simulink model "productionLine_5machines"  (R2024b)
settings: Solver=ode15s  StartTime=0.0  StopTime=100  FixedStep=0.1  RelTol=1e-3
model workspace (MAT data in the model file):
  bufferCapacity1 = 50
  bufferCapacity2 = 50
  bufferCapacity3 = 50
  bufferCapacity4 = 50
  bufferProcessedProducts = 50
  initialBufferCapacity = 100
undefined symbols (not defined in the file): m, n
libraries: rllib x1
settings Model: SimulationMode=accelerator  Creator=giopa  LastModifiedBy=giopa

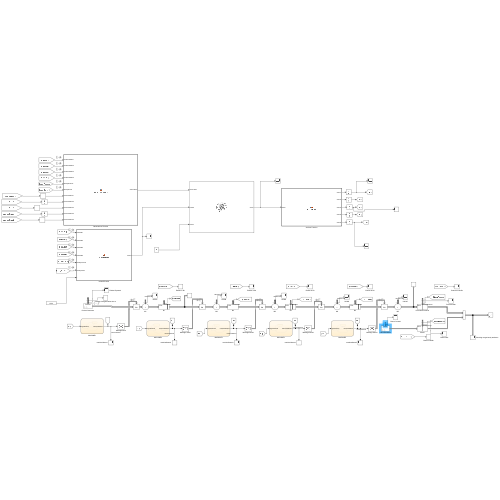
[thumbnail: Simulink's stored preview of the top-level diagram]
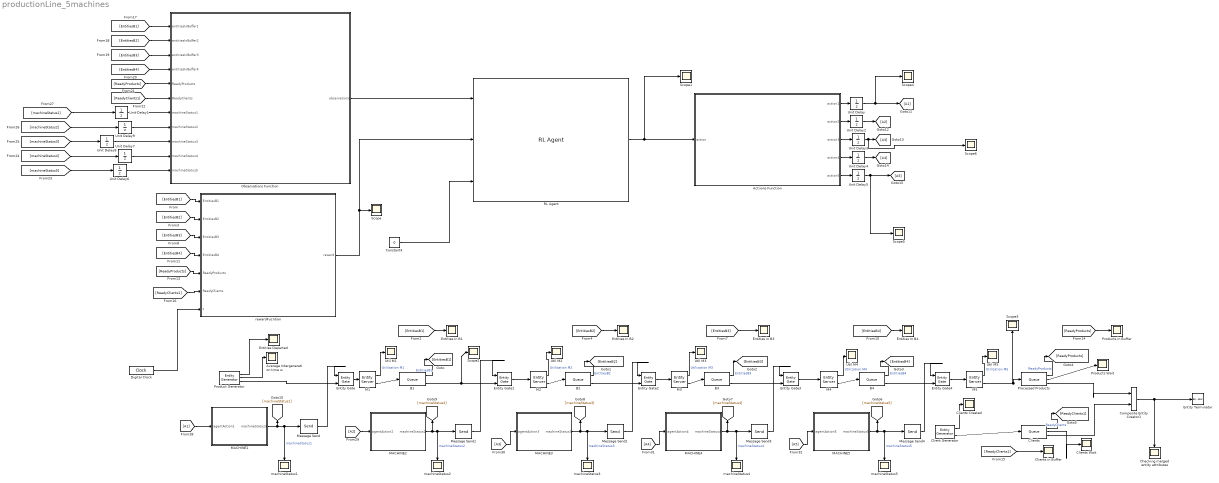
== system productionLine_5machines ==
  Actiions Function : MATLAB Function  TreatAsAtomicUnit=on
  Average Intergeneration time w : Scope
  B1 : Queue  InputPortMessageModes=m  OutputPortMessageModes=n,m  Capacity=bufferCapacity1  NumberEntitiesInBlock=on
      settings: OutputPortMap=o1,o5
  B2 : Queue  InputPortMessageModes=m  OutputPortMessageModes=n,m  Capacity=bufferCapacity2  NumberEntitiesInBlock=on
      settings: OutputPortMap=o1,o5
  B3 : Queue  InputPortMessageModes=m  OutputPortMessageModes=n,m  Capacity=bufferCapacity3  NumberEntitiesInBlock=on
      settings: OutputPortMap=o1,o5
  B4 : Queue  InputPortMessageModes=m  OutputPortMessageModes=n,m  Capacity=bufferCapacity4  NumberEntitiesInBlock=on
      settings: OutputPortMap=o1,o5
  Checking merged entity attributes : Scope
  Client Generator : EntityGenerator  OutputPortMessageModes=n,m  TimeSource=MATLAB action  IntergenerationTimeAction=|  GenerateEntityAtSimulationStart=off  GenerateAction=|  AttributeName=clientNumber  NumberEntitiesDeparted=on  EntityType=Structured  EntityTypeName=Client
      IntergenerationTimeAction=|
      | muI = 4.5;   % Mean intergeneration time 
      | dt = -muI * log(1 - rand());  % Exponential distribution
      GenerateAction=|
      | persistent clientNumber;
      | if isempty(clientNumber)
      |     clientNumber = 0; % Initialize the first client number
      | else
      |     clientNumber = clientNumber + 1; % Increment client number for each new entity
      | end
      | entity.clientNumber = clientNumber; % Assign the number to the entity's attribute
      settings: OutputPortMap=o0,o3
  "Clients " : Queue  InputPortMessageModes=m  OutputPortMessageModes=n,n,m  Capacity=50  NumberEntitiesInBlock=on  AverageWait=on
      settings: OutputPortMap=o1,o2,o5
  Clients Created : Scope
  Clients Wait : Scope
  Clients in Buffer : Scope
  Composite Entity Creator1 : CompositeEntityCreator  InputPortMessageModes=m,m  OutputPortMessageModes=m  EntityTypeName=Order  InputEntityName=Product|Client
      settings: InputPortMap=u0,u1
  Constant4 : Constant  Value=0
  Digital Clock : DigitalClock  SampleTime=0.1
  Entities Departed : Scope
  Entities In B1 : Scope
  Entities In B2 : Scope
  Entities In B4 : Scope
  Entities in B3 : Scope
  Entity Gate : EntityGate  InputPortMessageModes=m,m  OutputPortMessageModes=m  MatchingAttributeName=gateCheck  InitialValueOfMatchingAttribute=1  OpenGateAtSimulationStart=on
  Entity Gate{1..4} (4 alike) : EntityGate  InputPortMessageModes=m,m  OutputPortMessageModes=m  MatchingAttributeName=machineStatus  InitialValueOfMatchingAttribute=1
  Entity Terminator : EntityTerminator  InputPortMessageModes=m
  M{1..5} (5 alike) : EntityServer  InputPortMessageModes=m  OutputPortMessageModes=n,m  Capacity=1  ServiceTimeSource=Attribute  ServiceTimeValue=1  ServiceTimeAttributeName=processingTime  Utilization=on
      settings: OutputPortMap=o5,o9
  MACHINE1 : Stateflow chart  TreatAsAtomicUnit=on
  MACHINE2 : Stateflow chart  TreatAsAtomicUnit=on
  MACHINE3 : Stateflow chart  TreatAsAtomicUnit=on
  MACHINE4 : Stateflow chart  TreatAsAtomicUnit=on
  MACHINE5 : Stateflow chart  TreatAsAtomicUnit=on
  Message Send{,1..4} (5 alike) : Send  OutputPortMessageModes=m
  Observations Function : MATLAB Function  TreatAsAtomicUnit=on
  Processed Products : Queue  InputPortMessageModes=m  OutputPortMessageModes=n,n,m  Capacity=bufferProcessedProducts  NumberEntitiesInBlock=on  AverageWait=on
      settings: OutputPortMap=o1,o2,o5
  Product Generator : EntityGenerator  OutputPortMessageModes=n,n,m  Period=2.7  IntergenerationTimeAction=|  GenerateAction=|  ExitAction=|  AttributeName=processingTime|productNumber|entryTime  AttributeInitialValue=2|1|1  NumberEntitiesDeparted=on  AverageIntergenerationTime=on  EntityType=Structured  EntityTypeName=Product
      IntergenerationTimeAction=|
      | muI = 2;   % Mean intergeneration time 
      | dt = -muI * log(1 - rand());  % Exponential distribution
      GenerateAction=|
      | persistent rngInit;
      | if isempty(rngInit)
      |     seed = 12345;
      |     rng(seed);
      |     rngInit = true;
      | end
      | % Pattern: Exponential distribution
      | 
      | mu = 2;
      | entity.processingTime = -mu * log(1 - rand());
      | 
      | %assign productNumber aatribute to every entity
      | persistent productNumber
      | if isempty(productNumber)
      |     productNumber = 0;  
      | end
      | 
      | % Assign productNumber attribute
      | entity.productNumber = productNumber + 1; % Increment and assign the product number
      | productNumber = productNumber + 1;        % Update the product number for the next product
      ExitAction=|
      | persistent productNumber;
      | if isempty(productNumber)
      |     productNumber = 1; % Initialize the first client number
      | else
      |     productNumber = productNumber + 1; % Increment client number for each new entity
      | end
      | entity.productNumber = productNumber; % Assign the number to the entity's attribute
      settings: OutputPortMap=o0,o2,o3
  Products Wait : Scope
  Products in Buffer : Scope
  RL Agent : rllib/RL Agent  Agent=agent  ExternalActionAsInput=off  ProvideLastAction=off  ProvideCumRwd=off  TreatAsDirectFeedthrough=on  UseStrictObservationDataTypes=off
  Scope{,1..6} (7 alike) : Scope
  Unit Delay{,2..5} (5 alike) : UnitDelay  SampleTime=-1  HasFrameUpgradeWarning=on
  Unit Delay{1,6..9} (5 alike) : UnitDelay  InitialCondition=1  SampleTime=-1  HasFrameUpgradeWarning=on
  Util M{1..5} (5 alike) : Scope
  machineStatus{1..5} (5 alike) : Scope
  rewardFucntion : MATLAB Function  TreatAsAtomicUnit=on
  wires:
  Processed Products/2 -> Products Wait/1
  Entity Gate4/1 -> M5/1
  Product Generator/3 -> Entity Gate/2
  MACHINE3/1(machineStatus3) -> Message Send2/1, machineStatus3/1, [machineStatus3]  "machineStatus3"
  M1/1 -> Util M1/1  "Utilization M1"
  MACHINE1/1(machineStatus1) -> machineStatus1/1, Message Send/1, [machineStatus1]  "machineStatus1"
  MACHINE4/1(machineStatus4) -> Message Send3/1, machineStatus4/1, [machineStatus4]  "machineStatus4"
  MACHINE5/1(machineStatus5) -> Message Send4/1, machineStatus5/1, [machineStatus5]  "machineStatus5"
  B1/2 -> Scope2/1, Entity Gate1/2
  "Clients "/2 -> Clients Wait/1
  Product Generator/2 -> Average Intergeneration time w/1
  Processed Products/3 -> Composite Entity Creator1/1
  Client Generator/2 -> "Clients "/1
  M2/1 -> Util M2/1  "Utilization M2"
  Message Send3/1 -> Entity Gate3/1
  M4/1 -> Util M4/1  "Utilization M4"
  "Clients "/3 -> Composite Entity Creator1/2
  Entity Gate3/1 -> M4/1
  Entity Gate1/1 -> M2/1
  Entity Gate/1 -> M1/1
  Product Generator/1 -> Entities Departed/1
  M5/1 -> Util M5/1  "Utilization M5"
  Client Generator/1 -> Clients Created/1
  Composite Entity Creator1/1 -> Entity Terminator/1, Checking merged entity attributes/1
  B4/2 -> Entity Gate4/2
  M3/2 -> B3/1
  MACHINE2/1(machineStatus2) -> [machineStatus2], machineStatus2/1, Message Send1/1  "machineStatus2"
  Message Send2/1 -> Entity Gate2/1
  M3/1 -> Util M3/1  "Utilization M3"
  M4/2 -> B4/1
  B2/2 -> Entity Gate2/2
  Entity Gate2/1 -> M3/1
  Message Send4/1 -> Entity Gate4/1
  Message Send1/1 -> Entity Gate1/1
  M5/2 -> Processed Products/1, Scope3/1
  B3/2 -> Entity Gate3/2
  M2/2 -> B2/1
  Message Send/1 -> Entity Gate/1
  rewardFucntion/1(reward) -> Scope/1, RL Agent/2
  M1/2 -> B1/1
  B1/1 -> [EntitiesB1]  "EntitiesB1"
  [EntitiesB1] -> rewardFucntion/1(EntitiesB1)
  [EntitiesB1] -> Entities In B1/1
  B2/1 -> [EntitiesB2]  "EntitiesB2"
  [EntitiesB2] -> rewardFucntion/2(EntitiesB2)
  [EntitiesB2] -> Entities In B2/1
  B3/1 -> [EntitiesB3]  "EntitiesB3"
  [EntitiesB3] -> rewardFucntion/3(EntitiesB3)
  B4/1 -> [EntitiesB4]  "EntitiesB4"
  [EntitiesB4] -> Entities In B4/1
  [EntitiesB4] -> rewardFucntion/4(EntitiesB4)
  Processed Products/1 -> [ReadyProducts]  "ReadyProducts"
  [ReadyProducts] -> rewardFucntion/5(ReadyProducts)
  [ReadyProducts] -> Products in Buffer/1
  [ReadyClients1] -> rewardFucntion/6(ReadyClients)
  [EntitiesB3] -> Entities in B3/1
  [EntitiesB1] -> Observations Function/1(entitiesInBuffer1)
  [EntitiesB2] -> Observations Function/2(entitiesInBuffer2)
  [EntitiesB3] -> Observations Function/3(entitiesInBuffer3)
  "Clients "/1 -> [ReadyClients1]  "ReadyClients"
  [ReadyClients1] -> Clients in Buffer/1
  [ReadyProducts] -> Observations Function/5(ReadyProducts)
  [ReadyClients1] -> Observations Function/6(ReadyClients)
  [EntitiesB4] -> Observations Function/4(entitiesInBuffer4)
  [machineStatus5] -> Unit Delay6/1
  [machineStatus4] -> Unit Delay7/1
  [machineStatus3] -> Unit Delay8/1
  [machineStatus2] -> Unit Delay9/1
  [machineStatus1] -> Unit Delay1/1
  Observations Function/1(observations) -> RL Agent/1
  Constant4/1 -> RL Agent/3
  RL Agent/1 -> Scope1/1, Actiions Function/1(action)
  Actiions Function/1(action1) -> Unit Delay/1
  [A1] -> MACHINE1/1(agentAction1)
  Actiions Function/2(action2) -> Unit Delay2/1
  [A2] -> MACHINE2/1(agentAction2)
  Actiions Function/3(action3) -> Unit Delay3/1
  [A3] -> MACHINE3/1(agentAction3)
  Actiions Function/4(action4) -> Unit Delay4/1
  [A4] -> MACHINE4/1(agentAction4)
  Actiions Function/5(action5) -> Unit Delay5/1
  [A5] -> MACHINE5/1(agentAction5)
  Unit Delay/1 -> Scope4/1, [A1]
  Unit Delay1/1 -> Observations Function/7(machineStatus1)
  Unit Delay2/1 -> [A2]
  Unit Delay3/1 -> Scope6/1, [A3]
  Unit Delay4/1 -> [A4]
  Unit Delay5/1 -> Scope5/1, [A5]
  Unit Delay6/1 -> Observations Function/11(machineStatus5)
  Unit Delay7/1 -> Observations Function/10(machineStatus4)
  Unit Delay8/1 -> Observations Function/9(machineStatus3)
  Unit Delay9/1 -> Observations Function/8(machineStatus2)
  Digital Clock/1 -> rewardFucntion/7(t)

== stateflow chart productionLine_5machines/MACHINE5 ==
  state Failed
    entry:
    machineStatus5 = 0;
    repairTime5 = -meanRepairTime5 * log(1 - rand());
  state Idle
    entry:
    machineStatus5 = -1;
  state Working
    entry:
    machineStatus5 = 1;
    timeToFailure5 = -meanFailureTime5 * log(1 - rand());
  Working -> Failed [order 1] : [after(timeToFailure5, sec)]
  Failed -> Working : [after(repairTime5, sec)]
  (default) -> Working
  Idle -> Working : [agentAction5 == 1]
  Working -> Idle [order 2] : [agentAction5 == 0]
  data: meanRepairTime5 constant double =5; meanFailureTime5 constant double =50; machineStatus5 output; repairTime5 local; timeToFailure5 local; agentAction5 input

== matlab function productionLine_5machines/Observations Function ==
  data: entitiesInBuffer1 input; observations output; entitiesInBuffer2 input; entitiesInBuffer3 input; entitiesInBuffer4 input; ReadyProducts input; ReadyClients input; machineStatus1 input; machineStatus2 input; machineStatus3 input; machineStatus4 input; machineStatus5 input
function observations = gatherObservations(entitiesInBuffer1, entitiesInBuffer2, entitiesInBuffer3, ...
                                           entitiesInBuffer4, ReadyProducts, ReadyClients, ...
                                           machineStatus1, machineStatus2, machineStatus3, ...
                                           machineStatus4, machineStatus5)
    % Define maximum buffer capacity
    maxBufferCapacity = 50; 

    % Normalize buffer levels
    bufferLevels = [entitiesInBuffer1; entitiesInBuffer2; entitiesInBuffer3; entitiesInBuffer4] / maxBufferCapacity;

    % Normalize ready products and clients
    readyStates = [ReadyProducts; ReadyClients] / maxBufferCapacity;

    % Normalize machine states to [0, 1]
    machineStates = [machineStatus1; machineStatus2; machineStatus3; machineStatus4; machineStatus5];

    % Combine normalized observations into a single vector
    observations = [bufferLevels; readyStates; machineStates];
end

== matlab function productionLine_5machines/rewardFucntion ==
  data: EntitiesB1 input; EntitiesB2 input; EntitiesB3 input; EntitiesB4 input; ReadyProducts input; ReadyClients input; reward output; t input
function reward = calculateReward(EntitiesB1, EntitiesB2, EntitiesB3, EntitiesB4, ReadyProducts, ReadyClients, t)
    % Time tracking
    persistent lastTime
    if isempty(lastTime)
        lastTime = t;
        reward = 0;
        return;
    end

    % Calculate dt
    dt = t - lastTime;
    lastTime = t;

    % Cost weights
    bufferCost = 0.5;    % buffers 1,2,3,4
    productsCost = 1;  % readyProducts Buffer
    clientsCost = 1.3;   % readyClients Buffer

    % Calculate total cost
    totalCost = (EntitiesB1 * bufferCost + EntitiesB2 * bufferCost + EntitiesB3 * bufferCost + EntitiesB4 * bufferCost + ReadyProducts * productsCost + ReadyClients * clientsCost) * dt;



    % Total reward
    reward = -totalCost;
end

== matlab function productionLine_5machines/Actiions Function ==
  data: action input; action1 output; action2 output; action3 output; action4 output; action5 output
function [action1, action2, action3, action4, action5] = decodeAction(action)
    % Ensure action is treated as a numeric array
     % Directly use action as a numeric vector
    
    % Assign each binary digit to the respective machine's action
    action1 = action(1);
    action2 = action(2);
    action3 = action(3);
    action4 = action(4);
    action5 = action(5);
end

== stateflow chart productionLine_5machines/MACHINE2 ==
  state Failed
    entry:
    machineStatus2 = 0;
    repairTime2 = -meanRepairTime2 * log(1 - rand());
  state Idle
    entry:
    machineStatus2 = -1;
  state Working
    entry:
    machineStatus2 = 1;
    timeToFailure2 = -meanFailureTime2 * log(1 - rand());
  Working -> Failed [order 1] : [after(timeToFailure2, sec)]
  Failed -> Working : [after(repairTime2, sec)]
  (default) -> Working
  Idle -> Working : [agentAction2 == 1]
  Working -> Idle [order 2] : [agentAction2 == 0]
  data: meanRepairTime2 constant double =5; meanFailureTime2 constant double =50; machineStatus2 output; repairTime2 local; timeToFailure2 local; agentAction2 input

== stateflow chart productionLine_5machines/MACHINE3 ==
  state Failed
    entry:
    machineStatus3 = 0;
    repairTime3 = -meanRepairTime3 * log(1 - rand());
  state Idle
    entry:
    machineStatus3 = -1;
  state Working
    entry:
    machineStatus3 = 1;
    timeToFailure3 = -meanFailureTime3 * log(1 - rand());
  Working -> Failed [order 1] : [after(timeToFailure3, sec)]
  Failed -> Working : [after(repairTime3, sec)]
  (default) -> Working
  Idle -> Working : [agentAction3 == 1]
  Working -> Idle [order 2] : [agentAction3 == 0]
  data: meanRepairTime3 constant double =5; meanFailureTime3 constant double =50; machineStatus3 output; repairTime3 local; timeToFailure3 local; agentAction3 input

== stateflow chart productionLine_5machines/MACHINE1 ==
  state Failed
    entry:
    machineStatus1 = 0;
    repairTime1 = -meanRepairTime1 * log(1 - rand());
  state Idle
    entry:
    machineStatus1 = -1;
  state Working
    entry:
    machineStatus1 = 1;
    timeToFailure1 = -meanFailureTime1 * log(1 - rand());
  Working -> Failed [order 1] : [after(timeToFailure1, sec)]
  Failed -> Working : [after(repairTime1, sec)]
  (default) -> Working
  Idle -> Working : [agentAction1 == 1]
  Working -> Idle [order 2] : [agentAction1 == 0]
  data: meanRepairTime1 constant double =5; meanFailureTime1 constant double =50; machineStatus1 output; repairTime1 local; timeToFailure1 local; agentAction1 input

== stateflow chart productionLine_5machines/MACHINE4 ==
  state Failed
    entry:
    machineStatus4 = 0;
    repairTime4 = -meanRepairTime4 * log(1 - rand());
  state Idle
    entry:
    machineStatus4 = -1;
  state Working
    entry:
    machineStatus4 = 1;
    timeToFailure4 = -meanFailureTime4 * log(1 - rand());
  Working -> Failed [order 1] : [after(timeToFailure4, sec)]
  Failed -> Working : [after(repairTime4, sec)]
  (default) -> Working
  Idle -> Working : [agentAction4 == 1]
  Working -> Idle [order 2] : [agentAction4 == 0]
  data: meanRepairTime4 constant double =5; meanFailureTime4 constant double =50; machineStatus4 output; repairTime4 local; timeToFailure4 local; agentAction4 input
